simulink model "RL_Block_Lib"  (R2022b)
settings: Solver=FixedStepAuto  StartTime=0.0  StopTime=Inf  FixedStep=0.01  RelTol=1e-3
PostLoadFcn:
  | if any(exist('dsrtsu_mdlpostloadfcn', 'file') ~= 0), dsrtsu_mdlpostloadfcn('Execute', bdroot); end
InitFcn:
  | , if any(exist('dsmpb_private', 'file') ~= 0), dsmpb_private('dsmpb_mdlclblib', 'Init', bdroot); end,
values from neighbouring files (symbols this model uses):
  action_mean_selector_ppo = 1:num_actions    [ReinforcementLearningBlockInit.m]
  action_sampling_mode = 1    [ReinforcementLearningBlockInit.m]
  action_selector_ddpg = 1:num_actions    [ReinforcementLearningBlockInit.m]
  action_std_selector_ppo = 1:num_actions    [ReinforcementLearningBlockInit.m]
  action_type = 1    [ReinforcementLearningBlockInit.m]
  num_actions = 1    [ReinforcementLearningBlockInit.m]
  rl_algorithm = 1    [ReinforcementLearningBlockInit.m]
undefined symbols (not defined in the file or in its folder): NUMBER_OF_ACTIONS
libraries: simulink x3
PreSaveFcn:
  | , if any(exist('dsmpb_private', 'file') ~= 0), dsmpb_private('dsmpb_mdlclblib', 'PreSave', bdroot); end,
CloseFcn:
  | , if any(exist('dsmpb_private', 'file') ~= 0), dsmpb_private('dsmpb_mdlclblib', 'Close', bdroot); end,
settings Model: Creator=koch_luc  LastModifiedBy=kevin
settings SolverCC: AlgebraicLoopSolver=TrustRegion
settings OptimizationCC: BlockReduction=off  ConditionallyExecuteInputs=off  OptimizeBlockIOStorage=off  BufferReuse=off
settings DebuggingCC: TasksWithSamePriorityMsg=none  UnconnectedInputMsg=warning  UnconnectedOutputMsg=warning  UnconnectedLineMsg=warning  SFMachineParentedDataDiag=warning
settings HardwareCC: ProdBitPerPointer=32  ProdBitPerSizeT=32  ProdBitPerPtrDiffT=32  ProdLargestAtomicInteger=Integer  ProdWordSize=32  ProdLongLongMode=on  ProdHWDeviceType=Custom Processor->Custom
settings ModelReferenceCC: EnableRefExpFcnMdlSchedulingChecks=on  EnableParallelModelReferenceBuilds=on
settings SFSimCC: SimTargetLang=C++
settings RTWCC: Description=dSPACE Run-Time Target (for VEOS on Windows and ConfigurationDesk)  SystemTargetFile=dsrt.tlc  GenCodeOnly=on  MakeCommand=make_dsrt  TemplateMakefile=dsrt_default_tmf  RTWVerbose=off  TargetLang=C++
settings RTWCC: CustomSource=|
  | tensorflow/lite/micro/kernels/activations.cpp
  | tensorflow/lite/micro/kernels/activations_common.cpp
  | tensorflow/lite/micro/kernels/add.cpp
  | tensorflow/lite/micro/kernels/add_common.cpp
  | tensorflow/lite/micro/kernels/add_n.cpp
  | tensorflow/lite/micro/kernels/arg_min_max.cpp
  | tensorflow/lite/micro/kernels/assign_variable.cpp
  | tensorflow/lite/micro/kernels/batch_to_space_nd.cpp
  | tensorflow/lite/micro/kernels/broadcast_args.cpp
  | tensorflow/lite/micro/kernels/broadcast_to.cpp
  | tensorflow/lite/micro/kernels/call_once.cpp
  | tensorflow/lite/micro/kernels/cast.cpp
  | tensorflow/lite/micro/kernels/ceil.cpp
  | tensorflow/lite/micro/kernels/circular_buffer.cpp
  | tensorflow/lite/micro/kernels/circular_buffer_common.cpp
  | tensorflow/lite/micro/kernels/comparisons.cpp
  | tensorflow/lite/micro/kernels/concatenation.cpp
  | tensorflow/lite/micro/kernels/conv.cpp
  | tensorflow/lite/micro/kernels/conv_common.cpp
  | tensorflow/lite/micro/kernels/cumsum.cpp
  | tensorflow/lite/micro/kernels/depth_to_space.cpp
  | tensorflow/lite/micro/kernels/depthwise_conv.cpp
  | tensorflow/lite/micro/kernels/depthwise_conv_common.cpp
  | tensorflow/lite/micro/kernels/dequantize.cpp
  | tensorflow/lite/micro/kernels/dequantize_common.cpp
  | tensorflow/lite/micro/kernels/detection_postprocess.cpp
  | tensorflow/lite/micro/kernels/div.cpp
  | tensorflow/lite/micro/kernels/elementwise.cpp
  | tensorflow/lite/micro/kernels/elu.cpp
  | tensorflow/lite/micro/kernels/ethosu.cpp
  | tensorflow/lite/micro/kernels/exp.cpp
  | tensorflow/lite/micro/kernels/expand_dims.cpp
  | tensorflow/lite/micro/kernels/fill.cpp
  | tensorflow/lite/micro/kernels/floor.cpp
  | tensorflow/lite/micro/kernels/floor_div.cpp
  | tensorflow/lite/micro/kernels/floor_mod.cpp
  | tensorflow/lite/micro/kernels/fully_connected.cpp
  | tensorflow/lite/micro/kernels/fully_connected_common.cpp
  | tensorflow/lite/micro/kernels/gather.cpp
  | tensorflow/lite/micro/kernels/gather_nd.cpp
  | tensorflow/lite/micro/kernels/hard_swish.cpp
  | tensorflow/lite/micro/kernels/hard_swish_common.cpp
  | tensorflow/lite/micro/kernels/if.cpp
  | tensorflow/lite/micro/kernels/kernel_runner.cpp
  | tensorflow/lite/micro/kernels/kernel_util_micro.cpp
  | tensorflow/lite/micro/kernels/l2norm.cpp
  | tensorflow/lite/micro/kernels/l2_pool_2d.cpp
  | tensorflow/lite/micro/kernels/leaky_relu.cpp
  | tensorflow/lite/micro/kernels/leaky_relu_common.cpp
  | tensorflow/lite/micro/kernels/logical.cpp
  | tensorflow/lite/micro/kernels/logical_common.cpp
  | tensorflow/lite/micro/kernels/logistic.cpp
  | tensorflow/lite/micro/kernels/logistic_common.cpp
  | tensorflow/lite/micro/kernels/log_softmax.cpp
  | tensorflow/lite/micro/kernels/lstm_eval.cpp
  | tensorflow/lite/micro/kernels/maximum_minimum.cpp
  | tensorflow/lite/micro/kernels/micro_tensor_utils.cpp
  | tensorflow/lite/micro/kernels/mirror_pad.cpp
  | tensorflow/lite/micro/kernels/mul.cpp
  | tensorflow/lite/micro/kernels/mul_common.cpp
  | tensorflow/lite/micro/kernels/neg.cpp
  | tensorflow/lite/micro/kernels/pack.cpp
  | tensorflow/lite/micro/kernels/pad.cpp
  | tensorflow/lite/micro/kernels/pooling.cpp
  | tensorflow/lite/micro/kernels/pooling_common.cpp
  | tensorflow/lite/micro/kernels/prelu.cpp
  | tensorflow/lite/micro/kernels/prelu_common.cpp
  | tensorflow/lite/micro/kernels/quantize.cpp
  | tensorflow/lite/micro/kernels/quantize_common.cpp
  | tensorflow/lite/micro/kernels/read_variable.cpp
  | tensorflow/lite/micro/kernels/reduce.cpp
  | tensorflow/lite/micro/kernels/reduce_common.cpp
  | tensorflow/lite/micro/kernels/reshape.cpp
  | tensorflow/lite/micro/kernels/resize_bilinear.cpp
  | tensorflow/lite/micro/kernels/resize_nearest_neighbor.cpp
  | tensorflow/lite/micro/kernels/round.cpp
  | tensorflow/lite/micro/kernels/shape.cpp
  | tensorflow/lite/micro/kernels/slice.cpp
  | tensorflow/lite/micro/kernels/softmax.cpp
  | tensorflow/lite/micro/kernels/softmax_common.cpp
  | tensorflow/lite/micro/kernels/space_to_batch_nd.cpp
  | tensorflow/lite/micro/kernels/space_to_depth.cpp
  | tensorflow/lite/micro/kernels/split.cpp
  | tensorflow/lite/micro/kernels/split_v.cpp
  | tensorflow/lite/micro/kernels/squared_difference.cpp
  | tensorflow/lite/micro/kernels/squeeze.cpp
  | tensorflow/lite/micro/kernels/strided_slice.cpp
  | tensorflow/lite/micro/kernels/sub.cpp
  | tensorflow/lite/micro/kernels/sub_common.cpp
  | tensorflow/lite/micro/kernels/svdf.cpp
  | tensorflow/lite/micro/kernels/svdf_common.cpp
  | tensorflow/lite/micro/kernels/tanh.cpp
  | tensorflow/lite/micro/kernels/transpose.cpp
  | tensorflow/lite/micro/kernels/transpose_conv.cpp
  | tensorflow/lite/micro/kernels/unidirectional_sequence_lstm.cpp
  | tensorflow/lite/micro/kernels/unpack.cpp
  | tensorflow/lite/micro/kernels/var_handle.cpp
  | tensorflow/lite/micro/kernels/while.cpp
  | tensorflow/lite/micro/kernels/zeros_like.cpp
  | tensorflow/lite/core/api/flatbuffer_conversions.cpp
  | tensorflow/lite/core/api/op_resolver.cpp
  | tensorflow/lite/core/api/tensor_utils.cpp
  | tensorflow/lite/core/api/error_reporter.cpp
  | tensorflow/lite/schema/schema_utils.cpp
  | tensorflow/lite/kernels/kernel_util.cpp
  | tensorflow/lite/kernels/internal/reference/portable_tensor_utils.cpp
  | tensorflow/lite/kernels/internal/quantization_util.cpp
  | tensorflow/lite/c/common.cpp
  | tensorflow/lite/micro/memory_helpers.cpp
  | tensorflow/lite/micro/all_ops_resolver.cpp
  | tensorflow/lite/micro/micro_graph.cpp
  | tensorflow/lite/micro/micro_error_reporter.cpp
  | tensorflow/lite/micro/micro_context.cpp
  | tensorflow/lite/micro/micro_profiler.cpp
  | tensorflow/lite/micro/test_helpers.cpp
  | tensorflow/lite/micro/recording_micro_allocator.cpp
  | tensorflow/lite/micro/micro_interpreter.cpp
  | tensorflow/lite/micro/micro_time.cpp
  | tensorflow/lite/micro/micro_resource_variable.cpp
  | tensorflow/lite/micro/test_helper_custom_ops.cpp
  | tensorflow/lite/micro/flatbuffer_utils.cpp
  | tensorflow/lite/micro/mock_micro_graph.cpp
  | tensorflow/lite/micro/debug_log.cpp
  | tensorflow/lite/micro/micro_allocation_info.cpp
  | tensorflow/lite/micro/system_setup.cpp
  | tensorflow/lite/micro/micro_allocator.cpp
  | tensorflow/lite/micro/micro_string.cpp
  | tensorflow/lite/micro/micro_utils.cpp
  | tensorflow/lite/micro/fake_micro_context.cpp
  | tensorflow/lite/micro/arena_allocator/persistent_arena_buffer_allocator.cpp
  | tensorflow/lite/micro/arena_allocator/recording_single_arena_buffer_allocator.cpp
  | tensorflow/lite/micro/arena_allocator/non_persistent_arena_buffer_allocator.cpp
  | tensorflow/lite/micro/arena_allocator/single_arena_buffer_allocator.cpp
  | tensorflow/lite/micro/memory_planner/greedy_memory_planner.cpp
  | tensorflow/lite/micro/memory_planner/linear_memory_planner.cpp
  | tensorflow/lite/micro/memory_planner/non_persistent_buffer_planner_shim.cpp
settings STFCustomTargetCC: TargetLangStandard=C++03 (ISO)  ParMdlRefBuildCompliant=on  SystemTargetFile=dsrt.tlc
settings GRTTargetCC: TargetLangStandard=C++03 (ISO)  CompOptLevelCompliant=off  ConcurrentExecutionCompliant=off  CombineOutputUpdateFcns=off  MatFileLogging=off  CPPClassGenCompliant=off  UseToolchainInfoCompliant=off

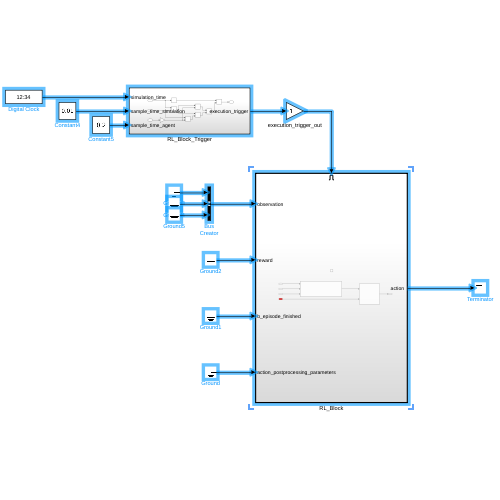
[thumbnail: Simulink's stored preview of the top-level diagram]
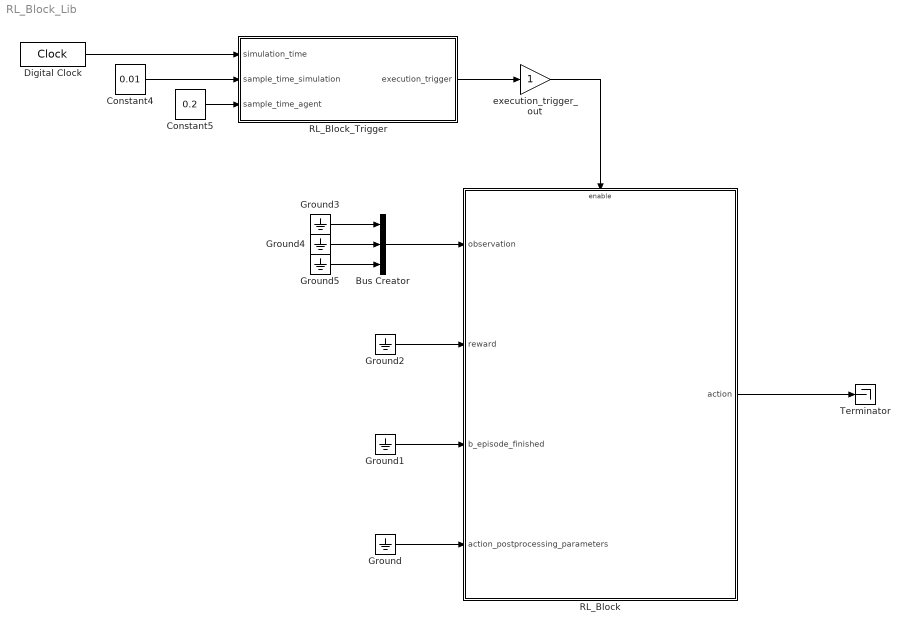
== system RL_Block_Lib ==
  Bus Creator : BusCreator  Inputs=3
  Constant4 : Constant  Value=0.01
  Constant5 : Constant  Value=0.2
  Digital Clock : DigitalClock  SampleTime=-1
  Ground{,1..5} (6 alike) : Ground
  RL_Block : Subsystem
  RL_Block_Trigger : Subsystem
  Terminator : Terminator
  execution_trigger_out : Gain  OutDataTypeStr=Inherit: Same as input
  wires:
  Ground1/1 -> RL_Block/3(b_episode_finished)
  Ground2/1 -> RL_Block/2(reward)
  Bus Creator/1 -> RL_Block/1(observation)
  RL_Block/1("action ") -> Terminator/1
  RL_Block_Trigger/1(execution_trigger) -> execution_trigger_out/1
  execution_trigger_out/1 -> RL_Block/Enable
  Digital Clock/1 -> RL_Block_Trigger/1(simulation_time)
  Constant4/1 -> RL_Block_Trigger/2(sample_time_simulation)
  Constant5/1 -> RL_Block_Trigger/3(sample_time_agent)
  Ground/1 -> RL_Block/4(action_postprocessing_parameters)
  Ground3/1 -> Bus Creator/1
  Ground4/1 -> Bus Creator/2
  Ground5/1 -> Bus Creator/3

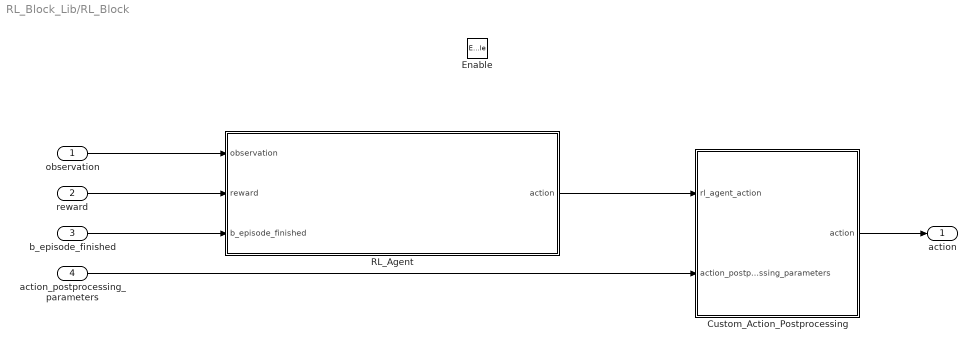
== system RL_Block_Lib/RL_Block ==
  observation : Inport
  reward : Inport  Port=2
  b_episode_finished : Inport  Port=3
  action_postprocessing_parameters : Inport  Port=4
  Enable : EnablePort
  Custom_Action_Postprocessing : Subsystem
  RL_Agent : Subsystem
  "action " : Outport
  wires:
  RL_Agent/1(action) -> Custom_Action_Postprocessing/1(rl_agent_action)
  action_postprocessing_parameters/1 -> Custom_Action_Postprocessing/2(action_postprocessing_parameters)
  b_episode_finished/1 -> RL_Agent/3(b_episode_finished)
  reward/1 -> RL_Agent/2(reward)
  observation/1 -> RL_Agent/1(observation)
  Custom_Action_Postprocessing/1("action ") -> "action "/1

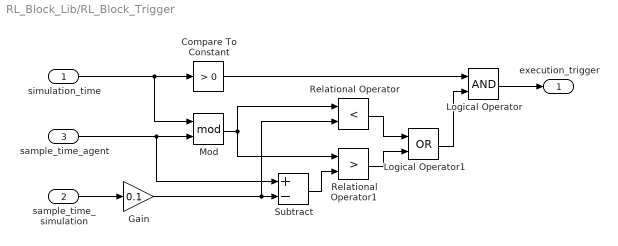
== system RL_Block_Lib/RL_Block_Trigger ==
  simulation_time : Inport
  sample_time_simulation : Inport  Port=2
  sample_time_agent : Inport  Port=3
  Compare To Constant : simulink/Logic and Bit Operations/Compare To Constant  relop=>  const=0  OutDataTypeStr=boolean
  Gain : Gain  Gain=0.1
  Logical Operator : Logic  AllPortsSameDT=off  OutDataTypeStr=boolean
  Logical Operator1 : Logic  Operator=OR  AllPortsSameDT=off  OutDataTypeStr=boolean
  Mod : Math  Operator=mod
  Relational Operator : RelationalOperator  Operator=<  OutDataTypeStr=boolean  RndMeth=Simplest  InputSameDT=off
  Relational Operator1 : RelationalOperator  Operator=>  OutDataTypeStr=boolean  RndMeth=Simplest  InputSameDT=off
  Subtract : Sum  Inputs=+-
  execution_trigger : Outport
  wires:
  simulation_time/1 -> Mod/1, Compare To Constant/1
  sample_time_agent/1 -> Subtract/1, Mod/2
  Mod/1 -> Relational Operator1/1, Relational Operator/1
  sample_time_simulation/1 -> Gain/1
  Logical Operator/1 -> execution_trigger/1
  Compare To Constant/1 -> Logical Operator/1
  Logical Operator1/1 -> Logical Operator/2
  Relational Operator/1 -> Logical Operator1/1
  Relational Operator1/1 -> Logical Operator1/2
  Gain/1 -> Relational Operator/2, Subtract/2
  Subtract/1 -> Relational Operator1/2

== system RL_Block_Lib/RL_Block/Custom_Action_Postprocessing ==
  rl_agent_action : Inport
  action_postprocessing_parameters : Inport  Port=2
  Terminator : Terminator
  "action " : Outport
  wires:
  rl_agent_action/1 -> "action "/1
  action_postprocessing_parameters/1 -> Terminator/1

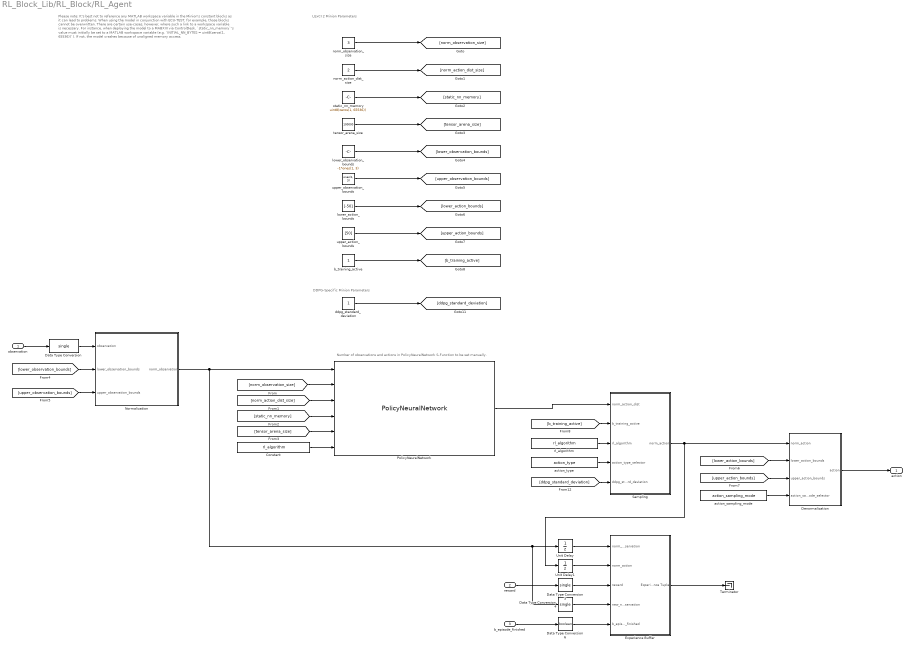
== system RL_Block_Lib/RL_Block/RL_Agent ==
  note: Please note:
      |
      | It's best not to reference any MATLAB workspace variable in the Minion's constant blocks as it can lead to
      | problems. When using the model in conjunction with ECU-TEST, for example, those blocks cannot be
      | overwritten.
      |
      | There are certain use-cases, however, where such a link to a workspace variable is necessary. For
      | instance, when deploying the model to a MABXIII via ControlDesk, `static_nn_memory`'s value must
      | initially be set to a MATLAB workspace variable (e.g. `INITIAL_NN_BYTES = uint8(zeros(1, 65536))`). If
      | not, the model crashes because of unaligned memory access.
  note: LExCI 2 Minion Parameters
  note: DDPG-Specific Minion Parameters
  note: Number of observations and actions in PolicyNeuralNetwork S-Function to be set manually.
  observation : Inport
  reward : Inport  Port=2
  b_episode_finished : Inport  Port=3
  Constant : Constant  Value=rl_algorithm  OutDataTypeStr=uint32
  Data Type Conversion : DataTypeConversion  OutDataTypeStr=single  SaturateOnIntegerOverflow=off  RndMeth=Floor
  Data Type Conversion3 : DataTypeConversion  OutDataTypeStr=single  SaturateOnIntegerOverflow=off  RndMeth=Floor
  Data Type Conversion4 : DataTypeConversion  OutDataTypeStr=single  SaturateOnIntegerOverflow=off  RndMeth=Floor
  Data Type Conversion6 : DataTypeConversion  OutDataTypeStr=boolean  SaturateOnIntegerOverflow=off  RndMeth=Floor
  Denormalization : Subsystem
  Experience Buffer : Subsystem
  Normalization : Subsystem
  PolicyNeuralNetwork : S-Function  InitFcn=try, set_param(gcb,'FunctionName','PolicyNeuralNetwork'), end  FunctionName=PolicyNeuralNetwork  SFunctionModules=PolicyNeuralNetwork_wrapper.cpp activations activations_common add add_common add_n arg_min_max assign_variable batch_to_space_nd broadcast_args broadcast_to call_once cast ceil circular_buffer circular_buffer_common comparisons concatenation conv conv_common cumsum depth_to_space depthwise_conv depthwise_conv_common dequantize dequantize_common detection_postprocess div elementwise elu ethosu exp expand_dims fill floor floor_div floor_mod fully_connected fully_connected_common gather gather_nd hard_swish hard_swish_common if kernel_runner kernel_util_micro l2norm l2_pool_2d leaky_relu leaky_relu_common logical logical_common logistic logistic_common log_softmax lstm_eval maximum_minimum micro_tensor_utils mirror_pad mul mul_common neg pack pad pooling pooling_common prelu prelu_common quantize quantize_common read_variable reduce reduce_common reshape resize_bilinear resize_nearest_neighbor round shape slice softmax softmax_common space_to_batch_nd space_to_depth split split_v squared_difference squeeze strided_slice sub sub_common svdf svdf_common tanh transpose transpose_conv unidirectional_sequence_lstm unpack var_handle while zeros_like flatbuffer_conversions op_resolver tensor_utils error_reporter schema_utils kernel_util portable_tensor_utils quantization_util common memory_helpers all_ops_resolver micro_graph micro_error_reporter micro_context micro_profiler test_helpers recording_micro_allocator micro_interpreter micro_time micro_resource_variable test_helper_custom_ops flatbuffer_utils mock_micro_graph debug_log micro_allocation_info system_setup micro_allocator micro_string micro_utils fake_micro_context persistent_arena_buffer_allocator recording_single_arena_buffer_allocator non_persistent_arena_buffer_allocator single_arena_buffer_allocator greedy_memory_planner linear_memory_planner non_persistent_buffer_planner_shim  SFunctionDeploymentMode=off  EnableBusSupport=off  mask(S-Function Builder){}
      mask help: Simulink:masks:SFunctionBuilder_MD
      mask init:
      | val = [[.9  0.75 0.75 1 1 .9 .9 1]',[1 1 0.75 0.75 .9 .9 1 .9]'];try , sys = get_param(gcb,'SfunBuilderFcnName');if isempty(sys), sys = get_param(gcb,'FunctionName'); end,catch, sys = get_param(gcb,'FunctionName'); end
      settings: CopyFcn=set_param(gcbh,'LinkStatus','none')  PreSaveFcn=try, set_param(gcb,'FunctionName','PolicyNeuralNetwork'), end  OpenFcn=sfunctionwizard(gcbh)
      mask Display:
      | plot(val(:,1),val(:,2))
      | disp(sys)
      | port_label('input',1,'norm_observation')
      | port_label('input',2,'norm_observation_size')
      | port_label('input',3,'norm_action_dist_size')
      | port_label('input',4,'static_nn_memory')
      | port_label('input',5,'tensor_arena_size')
      | port_label('input',6,'rl_algorithm')
      | port_label('output',1,'norm_action_dist')
  Sampling : Subsystem
  Terminator : Terminator
  Unit Delay : UnitDelay  InitialCondition=-1*ones(1,3)  SampleTime=-1  HasFrameUpgradeWarning=on
  Unit Delay1 : UnitDelay  InitialCondition=-1*ones(1,1)  SampleTime=-1  HasFrameUpgradeWarning=on
  action_sampling_mode : Constant  Value=action_sampling_mode  OutDataTypeStr=uint8
  action_type : Constant  Value=action_type  OutDataTypeStr=uint8
  b_training_active : Constant  OutDataTypeStr=boolean
  ddpg_standard_deviation : Constant  OutDataTypeStr=single
  lower_action_bounds : Constant  Value=[-50]  OutDataTypeStr=single
  lower_observation_bounds : Constant  Value=-1*ones(1, 3)  OutDataTypeStr=single
  norm_action_dist_size : Constant  Value=2  OutDataTypeStr=uint32
  norm_observation_size : Constant  Value=3  OutDataTypeStr=uint32
  rl_algorithm : Constant  Value=rl_algorithm  OutDataTypeStr=uint8
  static_nn_memory : Constant  Value=uint8(zeros(1, 65536))  OutDataTypeStr=uint8
  tensor_arena_size : Constant  Value=100000  OutDataTypeStr=uint32
  upper_action_bounds : Constant  Value=[50]  OutDataTypeStr=single
  upper_observation_bounds : Constant  Value=ones(1, 3)  OutDataTypeStr=single
  action : Outport
  wires:
  upper_action_bounds/1 -> [upper_action_bounds]
  PolicyNeuralNetwork/1 -> Sampling/1(norm_action_dist)
  upper_observation_bounds/1 -> [upper_observation_bounds]
  lower_action_bounds/1 -> [lower_action_bounds]
  [upper_observation_bounds] -> Normalization/3(upper_observation_bounds)
  [tensor_arena_size] -> PolicyNeuralNetwork/5
  b_episode_finished/1 -> Data Type Conversion6/1
  Unit Delay/1 -> Experience Buffer/1(norm_observation)
  [norm_observation_size] -> PolicyNeuralNetwork/2
  Data Type Conversion6/1 -> Experience Buffer/5(b_episode_finished)
  Unit Delay1/1 -> Experience Buffer/2(norm_action)
  Data Type Conversion3/1 -> Experience Buffer/3(reward)
  norm_observation_size/1 -> [norm_observation_size]
  Data Type Conversion/1 -> Normalization/1(observation)
  lower_observation_bounds/1 -> [lower_observation_bounds]
  Data Type Conversion4/1 -> Experience Buffer/4(new_norm_observation)
  reward/1 -> Data Type Conversion3/1
  norm_action_dist_size/1 -> [norm_action_dist_size]
  static_nn_memory/1 -> [static_nn_memory]
  Normalization/1(norm_observation) -> Unit Delay/1, Data Type Conversion4/1, PolicyNeuralNetwork/1
  observation/1 -> Data Type Conversion/1
  [norm_action_dist_size] -> PolicyNeuralNetwork/3
  [lower_observation_bounds] -> Normalization/2(lower_observation_bounds)
  tensor_arena_size/1 -> [tensor_arena_size]
  Experience Buffer/1(Experience Tuple) -> Terminator/1
  Sampling/1(norm_action) -> Unit Delay1/1, Denormalization/1(norm_action)
  Denormalization/1(action) -> action/1
  [lower_action_bounds] -> Denormalization/2(lower_action_bounds)
  [upper_action_bounds] -> Denormalization/3(upper_action_bounds)
  [static_nn_memory] -> PolicyNeuralNetwork/4
  b_training_active/1 -> [b_training_active]
  [b_training_active] -> Sampling/2(b_training_active)
  ddpg_standard_deviation/1 -> [ddpg_standard_deviation]
  action_sampling_mode/1 -> Denormalization/4(action_sampling_mode_selector)
  action_type/1 -> Sampling/4(action_type_selector)
  rl_algorithm/1 -> Sampling/3(rl_algorithm)
  [ddpg_standard_deviation] -> Sampling/5(ddpg_standard_deviation)
  Constant/1 -> PolicyNeuralNetwork/6

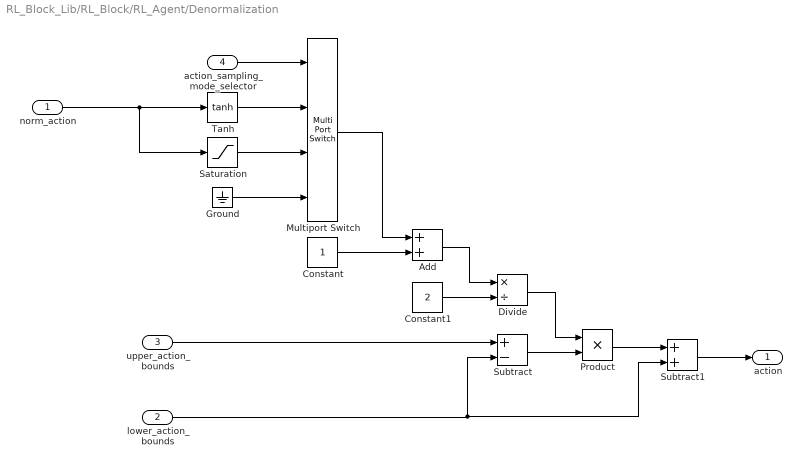
== system RL_Block_Lib/RL_Block/RL_Agent/Denormalization ==
  norm_action : Inport
  lower_action_bounds : Inport  Port=2
  upper_action_bounds : Inport  Port=3
  action_sampling_mode_selector : Inport  Port=4
  Add : Sum
  Constant : Constant  OutDataTypeStr=single
  Constant1 : Constant  Value=2  OutDataTypeStr=single
  Divide : Product  Inputs=*/
  Ground : Ground
  Multiport Switch : MultiPortSwitch  SaturateOnIntegerOverflow=off  InputSameDT=off
  Product : Product
  Saturation : Saturate  UpperLimit=1  LowerLimit=-1
  Subtract : Sum  Inputs=+-
  Subtract1 : Sum
  Tanh : Trigonometry  Operator=tanh
  action : Outport
  wires:
  action_sampling_mode_selector/1 -> Multiport Switch/1
  upper_action_bounds/1 -> Subtract/1
  Multiport Switch/1 -> Add/1
  lower_action_bounds/1 -> Subtract/2, Subtract1/2
  Add/1 -> Divide/1
  Subtract1/1 -> action/1
  Divide/1 -> Product/1
  Product/1 -> Subtract1/1
  Constant1/1 -> Divide/2
  Constant/1 -> Add/2
  Tanh/1 -> Multiport Switch/2
  Subtract/1 -> Product/2
  norm_action/1 -> Saturation/1, Tanh/1
  Saturation/1 -> Multiport Switch/3
  Ground/1 -> Multiport Switch/4

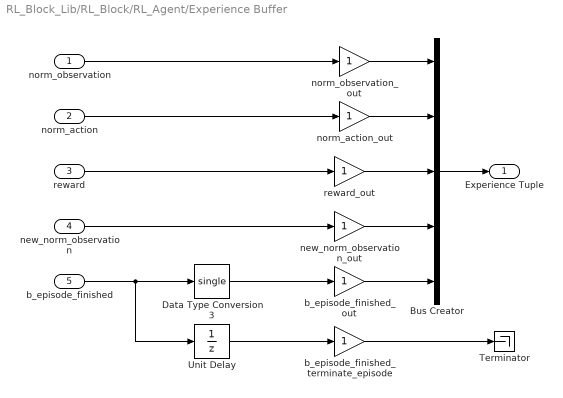
== system RL_Block_Lib/RL_Block/RL_Agent/Experience Buffer ==
  norm_observation : Inport
  norm_action : Inport  Port=2
  reward : Inport  Port=3
  new_norm_observation : Inport  Port=4
  b_episode_finished : Inport  Port=5
  Bus Creator : BusCreator  Inputs=5
  Data Type Conversion3 : DataTypeConversion  OutDataTypeStr=single  SaturateOnIntegerOverflow=off  RndMeth=Floor
  Terminator : Terminator
  Unit Delay : UnitDelay  SampleTime=-1  HasFrameUpgradeWarning=on
  b_episode_finished_out : Gain  OutDataTypeStr=Inherit: Same as input
  b_episode_finished_terminate_episode : Gain  OutDataTypeStr=Inherit: Same as input
  new_norm_observation_out : Gain  OutDataTypeStr=Inherit: Same as input
  norm_action_out : Gain  OutDataTypeStr=Inherit: Same as input
  norm_observation_out : Gain  OutDataTypeStr=Inherit: Same as input
  reward_out : Gain  OutDataTypeStr=Inherit: Same as input
  Experience Tuple : Outport
  wires:
  b_episode_finished_terminate_episode/1 -> Terminator/1
  Unit Delay/1 -> b_episode_finished_terminate_episode/1
  b_episode_finished_out/1 -> Bus Creator/5
  reward_out/1 -> Bus Creator/3
  norm_action_out/1 -> Bus Creator/2
  norm_observation_out/1 -> Bus Creator/1
  Data Type Conversion3/1 -> b_episode_finished_out/1
  Bus Creator/1 -> Experience Tuple/1
  b_episode_finished/1 -> Data Type Conversion3/1, Unit Delay/1
  reward/1 -> reward_out/1
  norm_action/1 -> norm_action_out/1
  norm_observation/1 -> norm_observation_out/1
  new_norm_observation/1 -> new_norm_observation_out/1
  new_norm_observation_out/1 -> Bus Creator/4

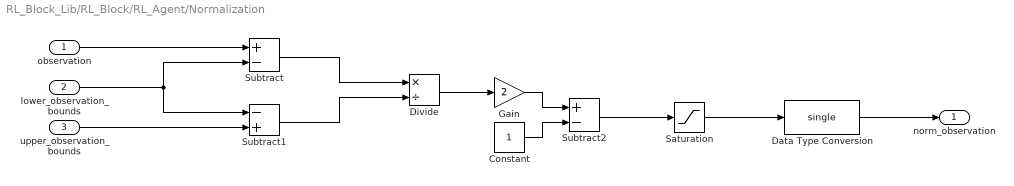
== system RL_Block_Lib/RL_Block/RL_Agent/Normalization ==
  observation : Inport
  lower_observation_bounds : Inport  Port=2
  upper_observation_bounds : Inport  Port=3
  Constant : Constant
  Data Type Conversion : DataTypeConversion  OutDataTypeStr=single  SaturateOnIntegerOverflow=off  RndMeth=Floor
  Divide : Product  Inputs=*/
  Gain : Gain  Gain=2
  Saturation : Saturate  UpperLimit=1  LowerLimit=-1
  Subtract : Sum  Inputs=+-
  Subtract1 : Sum  Inputs=-+
  Subtract2 : Sum  Inputs=+-
  norm_observation : Outport
  wires:
  Saturation/1 -> Data Type Conversion/1
  lower_observation_bounds/1 -> Subtract1/1, Subtract/2
  upper_observation_bounds/1 -> Subtract1/2
  observation/1 -> Subtract/1
  Data Type Conversion/1 -> norm_observation/1
  Divide/1 -> Gain/1
  Subtract1/1 -> Divide/2
  Subtract/1 -> Divide/1
  Gain/1 -> Subtract2/1
  Subtract2/1 -> Saturation/1
  Constant/1 -> Subtract2/2

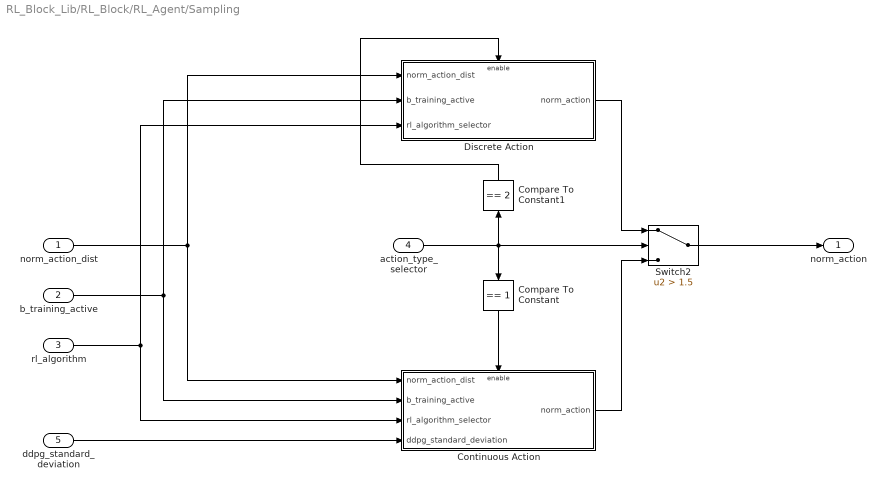
== system RL_Block_Lib/RL_Block/RL_Agent/Sampling ==
  norm_action_dist : Inport
  b_training_active : Inport  Port=2
  rl_algorithm : Inport  Port=3
  action_type_selector : Inport  Port=4
  ddpg_standard_deviation : Inport  Port=5
  Compare To Constant : simulink/Logic and Bit Operations/Compare To Constant  relop===  const=1  OutDataTypeStr=boolean
  Compare To Constant1 : simulink/Logic and Bit Operations/Compare To Constant  relop===  const=2  OutDataTypeStr=boolean
  Continuous Action : Subsystem
  Discrete Action : Subsystem
  Switch2 : Switch  Criteria=u2 > Threshold  Threshold=1.5  SaturateOnIntegerOverflow=off  InputSameDT=off
  norm_action : Outport
  wires:
  Continuous Action/1("norm_action ") -> Switch2/3
  Switch2/1 -> norm_action/1
  Compare To Constant/1 -> Continuous Action/Enable
  norm_action_dist/1 -> Continuous Action/1(norm_action_dist), Discrete Action/1(norm_action_dist)
  action_type_selector/1 -> Compare To Constant1/1, Compare To Constant/1, Switch2/2
  Compare To Constant1/1 -> Discrete Action/Enable
  Discrete Action/1("norm_action ") -> Switch2/1
  b_training_active/1 -> Continuous Action/2(b_training_active), Discrete Action/2(b_training_active)
  rl_algorithm/1 -> Discrete Action/3(rl_algorithm_selector), Continuous Action/3(rl_algorithm_selector)
  ddpg_standard_deviation/1 -> Continuous Action/4(ddpg_standard_deviation)

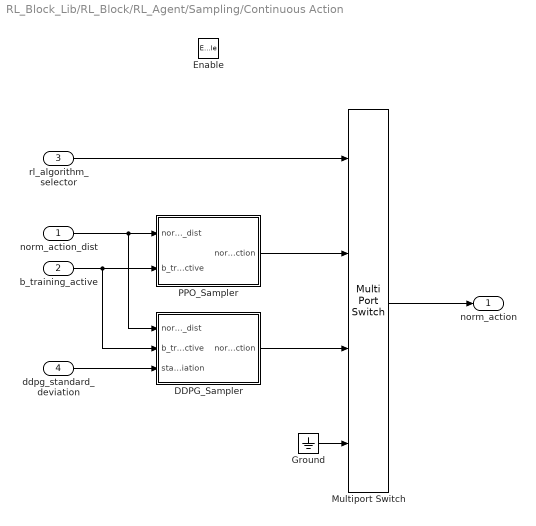
== system RL_Block_Lib/RL_Block/RL_Agent/Sampling/Continuous Action ==
  norm_action_dist : Inport
  b_training_active : Inport  Port=2
  rl_algorithm_selector : Inport  Port=3
  ddpg_standard_deviation : Inport  Port=4
  Enable : EnablePort
  DDPG_Sampler : Subsystem
  Ground : Ground
  Multiport Switch : MultiPortSwitch  SaturateOnIntegerOverflow=off  InputSameDT=off
  PPO_Sampler : Subsystem
  "norm_action " : Outport
  wires:
  rl_algorithm_selector/1 -> Multiport Switch/1
  norm_action_dist/1 -> DDPG_Sampler/1(norm_action_dist), PPO_Sampler/1(norm_action_dist)
  b_training_active/1 -> PPO_Sampler/2(b_training_active), DDPG_Sampler/2(b_training_active)
  PPO_Sampler/1("norm_action ") -> Multiport Switch/2
  ddpg_standard_deviation/1 -> DDPG_Sampler/3(standard_deviation)
  DDPG_Sampler/1("norm_action ") -> Multiport Switch/3
  Ground/1 -> Multiport Switch/4
  Multiport Switch/1 -> "norm_action "/1

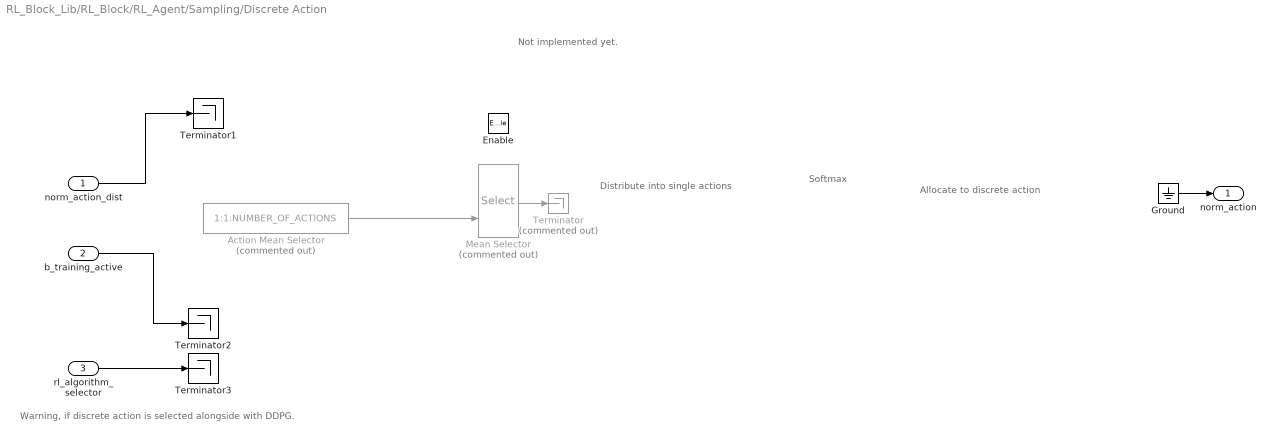
== system RL_Block_Lib/RL_Block/RL_Agent/Sampling/Discrete Action ==
  note: Distribute into single actions
  note: Softmax
  note: Allocate to discrete action
  note: Warning, if discrete action is selected alongside with DDPG.
  note: Not implemented yet.
  norm_action_dist : Inport
  b_training_active : Inport  Port=2
  rl_algorithm_selector : Inport  Port=3
  Enable : EnablePort
  Action Mean Selector : Constant  Commented=on  Value=1:1:NUMBER_OF_ACTIONS  OutDataTypeStr=single
  Ground : Ground
  Mean Selector : Selector  Commented=on  InputPortWidth=2*NUMBER_OF_ACTIONS  IndexOptions=Index vector (port)  Indices=1  OutputSizes=1
  Terminator : Terminator  Commented=on
  Terminator1 : Terminator
  Terminator2 : Terminator
  Terminator3 : Terminator
  "norm_action " : Outport
  wires:
  Action Mean Selector/1 -> Mean Selector/2
  norm_action_dist/1 -> Terminator1/1
  Mean Selector/1 -> Terminator/1
  Ground/1 -> "norm_action "/1
  b_training_active/1 -> Terminator2/1
  rl_algorithm_selector/1 -> Terminator3/1

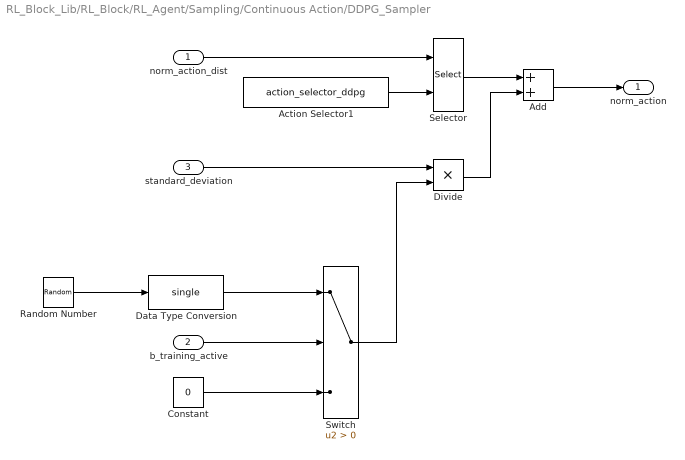
== system RL_Block_Lib/RL_Block/RL_Agent/Sampling/Continuous Action/DDPG_Sampler ==
  norm_action_dist : Inport
  b_training_active : Inport  Port=2
  standard_deviation : Inport  Port=3
  Action Selector1 : Constant  Value=action_selector_ddpg  OutDataTypeStr=single
  Add : Sum
  Constant : Constant  Value=0  OutDataTypeStr=single
  Data Type Conversion : DataTypeConversion  OutDataTypeStr=single  SaturateOnIntegerOverflow=off  RndMeth=Floor
  Divide : Product  Inputs=**
  Random Number : RandomNumber  Mean=zeros(1,num_actions)  Variance=ones(1,num_actions)  Seed=randi(1000,1,num_actions)
  Selector : Selector  IndexOptions=Index vector (port)  Indices=1  OutputSizes=1
  Switch : Switch  Criteria=u2 > Threshold  SaturateOnIntegerOverflow=off  InputSameDT=off
  "norm_action " : Outport
  wires:
  Switch/1 -> Divide/2
  standard_deviation/1 -> Divide/1
  b_training_active/1 -> Switch/2
  Constant/1 -> Switch/3
  Random Number/1 -> Data Type Conversion/1
  Add/1 -> "norm_action "/1
  Data Type Conversion/1 -> Switch/1
  norm_action_dist/1 -> Selector/1
  Divide/1 -> Add/2
  Action Selector1/1 -> Selector/2
  Selector/1 -> Add/1

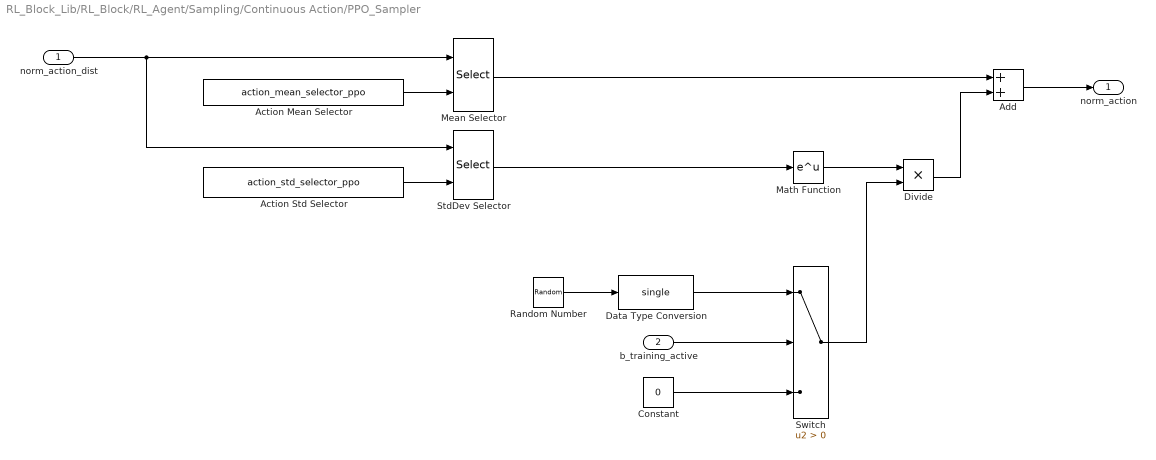
== system RL_Block_Lib/RL_Block/RL_Agent/Sampling/Continuous Action/PPO_Sampler ==
  norm_action_dist : Inport
  b_training_active : Inport  Port=2
  Action Mean Selector : Constant  Value=action_mean_selector_ppo  OutDataTypeStr=single
  Action Std Selector : Constant  Value=action_std_selector_ppo  OutDataTypeStr=single
  Add : Sum
  Constant : Constant  Value=0  OutDataTypeStr=single
  Data Type Conversion : DataTypeConversion  OutDataTypeStr=single  SaturateOnIntegerOverflow=off  RndMeth=Floor
  Divide : Product  Inputs=**
  Math Function : Math
  Mean Selector : Selector  IndexOptions=Index vector (port)  Indices=1  OutputSizes=1
  Random Number : RandomNumber  Mean=zeros(1,num_actions)  Variance=ones(1,num_actions)  Seed=randi(1000,1,num_actions)
  StdDev Selector : Selector  IndexOptions=Index vector (port)  Indices=2  OutputSizes=1
  Switch : Switch  Criteria=u2 > Threshold  SaturateOnIntegerOverflow=off  InputSameDT=off
  "norm_action " : Outport
  wires:
  Divide/1 -> Add/2
  Mean Selector/1 -> Add/1
  Data Type Conversion/1 -> Switch/1
  Add/1 -> "norm_action "/1
  StdDev Selector/1 -> Math Function/1
  Random Number/1 -> Data Type Conversion/1
  Action Mean Selector/1 -> Mean Selector/2
  Constant/1 -> Switch/3
  b_training_active/1 -> Switch/2
  Math Function/1 -> Divide/1
  Action Std Selector/1 -> StdDev Selector/2
  Switch/1 -> Divide/2
  norm_action_dist/1 -> StdDev Selector/1, Mean Selector/1
